simulink model "two_states_three_transitions"  (R2017b)
settings: Solver=FixedStepDiscrete  StartTime=0.0  StopTime=10.0  RelTol=1e-3
settings Model: Creator=flosch  LastModifiedBy=flosch
settings ConfigComp: CovScope=ReferencedModels  CovIncludeTopModel=off

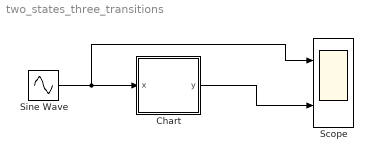
== system two_states_three_transitions ==
  Chart : Stateflow chart  TreatAsAtomicUnit=on
  Scope : Scope  NumInputPorts=2
  Sine Wave : Sin  SampleTime=0
  wires:
  Sine Wave/1 -> Scope/1, Chart/1(x)
  Chart/1(y) -> Scope/2

== stateflow chart two_states_three_transitions/Chart ==
  note: cyc = 5
      | obj = 6
      | lines = 5
  state Potato
    entry: y = x;
  state Kitten
    entry: y = 0;
  (default) -> Potato
  Kitten -> Potato : [x < t0]
  Potato -> Kitten [order 2] : [x == t0]
  Potato -> Kitten [order 1] : [x > t0]
  data: t0 constant double =0.0; x input; y output
